simulink library "Dampers_Independent"  (R2020a)
settings: Solver=VariableStepAuto  StartTime=0.0  StopTime=10.0  RelTol=1e-3
libraries: sm_car_lib x6, fl_lib x6
Description:
  | Component of Simscape Vehicle Templates Library
  | 
  | Copyright 2018-2020 The MathWorks, Inc.
settings Model: Creator=smiller  LastModifiedBy=smiller
settings DataIOCC: ReturnWorkspaceOutputs=off
settings DebuggingCC: ArithmeticOperatorsInVariantConditions=warning
settings SFSimCC: CustomCodeUndefinedFunction=UseInterfaceOnly

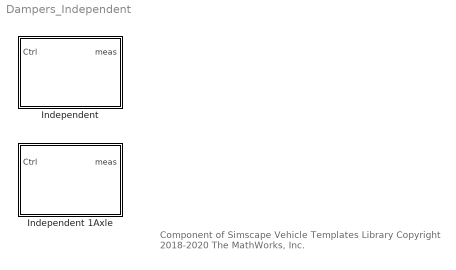
== system Dampers_Independent ==
  note: Component of Simscape Vehicle Templates Library
      | Copyright 2018-2020 The MathWorks, Inc.
  Independent : Subsystem  VariantControl=Independent  mask(Independent Dampers){InitTriggerDropdown=0}
      mask prompts: InitTriggerDropdown "Initialization Trigger Dropdown"
      mask help: Dampers with no physical connections.
      mask init:
      | curblk = gcb;
      | 
      | % Trigger Mask Initialization for 
      | % variant subsystems below this level
      | sm_car_lib_maskInitTrigger(curblk);
      mask TypeOptions InitTriggerDropdown: 0 | 1
  Independent 1Axle : Subsystem  VariantControl=Independent  mask(Independent Dampers){InitTriggerDropdown=0}
      mask prompts: InitTriggerDropdown "Initialization Trigger Dropdown"
      mask help: Dampers with no physical connections.
      mask init:
      | curblk = gcb;
      | 
      | % Trigger Mask Initialization for 
      | % variant subsystems below this level
      | sm_car_lib_maskInitTrigger(curblk);
      mask TypeOptions InitTriggerDropdown: 0 | 1

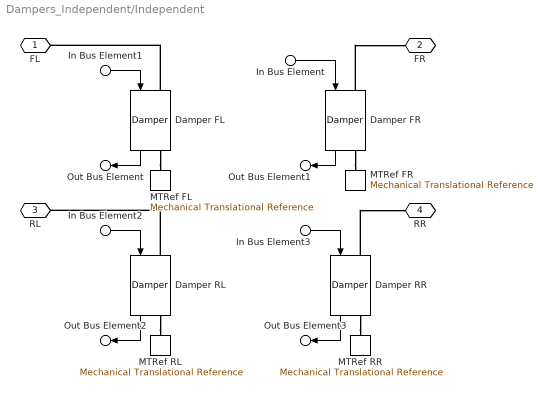
== system Dampers_Independent/Independent ==
  In Bus Element1 : Inport  PortName=Ctrl  Element=FL
  In Bus Element : Inport  PortName=Ctrl  Element=FR
  In Bus Element2 : Inport  PortName=Ctrl  Element=RL
  In Bus Element3 : Inport  PortName=Ctrl  Element=RR
  Damper FL : sm_car_lib/Springs Dampers/Damper  VariantControl=Variant1  LabelModeActiveChoice=Linear  Damper=Damper.Front  VariantLabel=Damper.Front.class.Value  InitTriggerDropdown=0
      settings: AttributesFormatString=%<ActiveVariant>
  Damper FR : sm_car_lib/Springs Dampers/Damper  VariantControl=Variant1  LabelModeActiveChoice=Linear  Damper=Damper.Front  VariantLabel=Damper.Front.class.Value  InitTriggerDropdown=0
      settings: AttributesFormatString=%<ActiveVariant>
  Damper RL : sm_car_lib/Springs Dampers/Damper  VariantControl=Variant1  LabelModeActiveChoice=Linear  Damper=Damper.Rear  VariantLabel=Damper.Rear.class.Value  InitTriggerDropdown=0
      settings: AttributesFormatString=%<ActiveVariant>
  Damper RR : sm_car_lib/Springs Dampers/Damper  VariantControl=Variant1  LabelModeActiveChoice=Linear  Damper=Damper.Rear  VariantLabel=Damper.Rear.class.Value  InitTriggerDropdown=0
      settings: AttributesFormatString=%<ActiveVariant>
  MTRef FL : fl_lib/Mechanical/Translational Elements/Mechanical Translational Reference
  MTRef FR : fl_lib/Mechanical/Translational Elements/Mechanical Translational Reference
  MTRef RL : fl_lib/Mechanical/Translational Elements/Mechanical Translational Reference
  MTRef RR : fl_lib/Mechanical/Translational Elements/Mechanical Translational Reference
  FL : PMIOPort  Side=Left
  FR : PMIOPort  Port=2  Side=Right
  RL : PMIOPort  Port=3  Side=Left
  RR : PMIOPort  Port=4  Side=Right
  Out Bus Element : Outport  VectorParamsAs1DForOutWhenUnconnected=off  PortName=meas  Element=FL
  Out Bus Element1 : Outport  VectorParamsAs1DForOutWhenUnconnected=off  PortName=meas  Element=FR
  Out Bus Element2 : Outport  VectorParamsAs1DForOutWhenUnconnected=off  PortName=meas  Element=RL
  Out Bus Element3 : Outport  VectorParamsAs1DForOutWhenUnconnected=off  PortName=meas  Element=RR
  wires:
  Damper RR/1 -> Out Bus Element3/1
  Damper RL/1 -> Out Bus Element2/1
  In Bus Element2/1 -> Damper RL/1
  In Bus Element3/1 -> Damper RR/1
  Damper FR/1 -> Out Bus Element1/1
  Damper FL/1 -> Out Bus Element/1
  In Bus Element1/1 -> Damper FL/1
  In Bus Element/1 -> Damper FR/1
  connections:
  Damper FL/RConn1 -- MTRef FL/LConn1
  Damper FL/LConn1 -- FL/RConn1
  Damper RL/RConn1 -- MTRef RL/LConn1
  Damper RL/LConn1 -- RL/RConn1
  Damper RR/RConn1 -- MTRef RR/LConn1
  Damper RR/LConn1 -- RR/RConn1
  Damper FR/RConn1 -- MTRef FR/LConn1
  Damper FR/LConn1 -- FR/RConn1

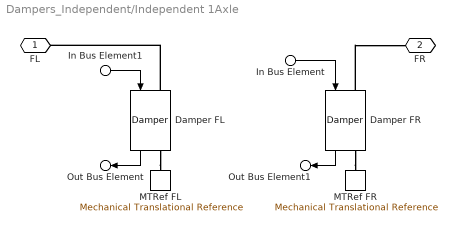
== system Dampers_Independent/Independent 1Axle ==
  In Bus Element1 : Inport  PortName=Ctrl  Element=FL
  In Bus Element : Inport  PortName=Ctrl  Element=FR
  Damper FL : sm_car_lib/Springs Dampers/Damper  VariantControl=Variant1  LabelModeActiveChoice=Linear  Damper=Damper.Front  VariantLabel=Damper.Front.class.Value  InitTriggerDropdown=0
      settings: AttributesFormatString=%<ActiveVariant>
  Damper FR : sm_car_lib/Springs Dampers/Damper  VariantControl=Variant1  LabelModeActiveChoice=Linear  Damper=Damper.Front  VariantLabel=Damper.Front.class.Value  InitTriggerDropdown=0
      settings: AttributesFormatString=%<ActiveVariant>
  MTRef FL : fl_lib/Mechanical/Translational Elements/Mechanical Translational Reference
  MTRef FR : fl_lib/Mechanical/Translational Elements/Mechanical Translational Reference
  FL : PMIOPort  Side=Left
  FR : PMIOPort  Port=2  Side=Right
  Out Bus Element : Outport  VectorParamsAs1DForOutWhenUnconnected=off  PortName=meas  Element=FL
  Out Bus Element1 : Outport  VectorParamsAs1DForOutWhenUnconnected=off  PortName=meas  Element=FR
  wires:
  In Bus Element/1 -> Damper FR/1
  In Bus Element1/1 -> Damper FL/1
  Damper FL/1 -> Out Bus Element/1
  Damper FR/1 -> Out Bus Element1/1
  connections:
  Damper FR/LConn1 -- FR/RConn1
  Damper FR/RConn1 -- MTRef FR/LConn1
  Damper FL/LConn1 -- FL/RConn1
  Damper FL/RConn1 -- MTRef FL/LConn1
